simulink model "s0526"  (Simulink 6.0)
settings: Solver=ode45  SolverMode=SingleTasking  StartTime=0.0  StopTime=999999  MaxStep=10  RelTol=1e-3  AbsTol=1e-6
values from neighbouring files (symbols this model uses):
  Kps = 1    [m0305.m]    (also in m0306.m; m0311.m; m0313.m; m0314.m = 0.143)
  T1 = 3*T1    (= 0.3)    [m0203.m]    (also in m0204.m = 0.1; m0205.m = 0.1; m0207.m = 0.1; m0221d.m = 1/a0)
undefined symbols (not defined in the file or in its folder): Kir
settings Model: LastModifiedBy=Froriep
settings DataIOCC: LimitDataPoints=off  SaveOutput=off  SaveTime=off
settings OptimizationCC: BooleanDataType=off
settings DebuggingCC: SolverPrmCheckMsg=none
settings HardwareCC: TargetUnknown=on
settings STFCustomTargetCC: TargetFcnLib=ansi_tfl_tmw.mat  GenFloatMathFcnCalls=ANSI_C  ModelReferenceCompliant=off  SystemTargetFile=grt.tlc

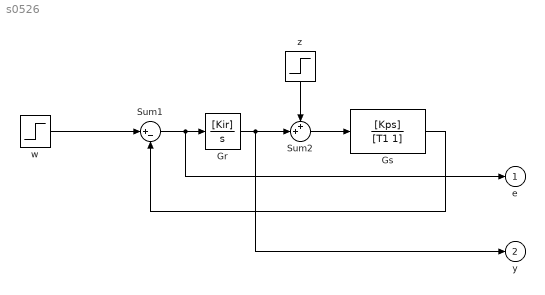
== system s0526 ==
  Gr : TransferFcn  Numerator=[Kir]  Denominator=[1 0]
  Gs : TransferFcn  Numerator=[Kps]  Denominator=[T1 1]
  Sum1 : Sum  Inputs=|+-  SaturateOnIntegerOverflow=on  InputSameDT=on
  Sum2 : Sum  Inputs=++|  SaturateOnIntegerOverflow=on  InputSameDT=on
  w : Step  After=0  SampleTime=0
  z : Step  Orientation=down  Time=0  SampleTime=0
  e : Outport
  y : Outport  Port=2
  wires:
  Gr/1 -> y/1, Sum2/2
  Sum1/1 -> e/1, Gr/1
  w/1 -> Sum1/1
  Gs/1 -> Sum1/2
  Sum2/1 -> Gs/1
  z/1 -> Sum2/1
